simulink model "Progetto_a1_simulink_non_lineare"  (R2022b)
settings: Solver=VariableStepAuto  StartTime=0.0  StopTime=100  RelTol=1e-3
values from neighbouring files (symbols this model uses):
  DD_ampiezza = 0.3    [Progetto_a1.m]
  DD_frequenza = 0.025    [Progetto_a1.m]
  denR = deR{1}    [Progetto_a1.m]
  NN_ampiezza = 0.2    [Progetto_a1.m]
  NN_frequenza = 1e3    (= 1000)    [Progetto_a1.m]
  numR = nuR{1}    [Progetto_a1.m]
  u_e = 2.17    [Progetto_a1.m]
  WW = 2    [Progetto_a1.m]
  x = [1,2,3,4]    [Progetto_a1.m]
  x01 = theta_e    (= 1.0471975512)    [Progetto_a1.m]
  x02 = 0    [Progetto_a1.m]
  ye = x01    (= 1.0471975512)    [Progetto_a1.m]
settings Model: Creator=anton  LastModifiedBy=anton

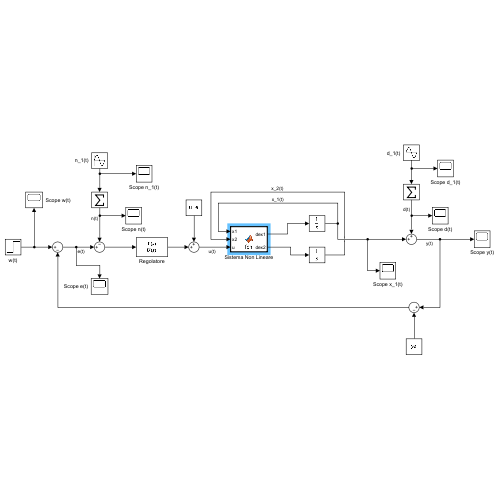
[thumbnail: Simulink's stored preview of the top-level diagram]
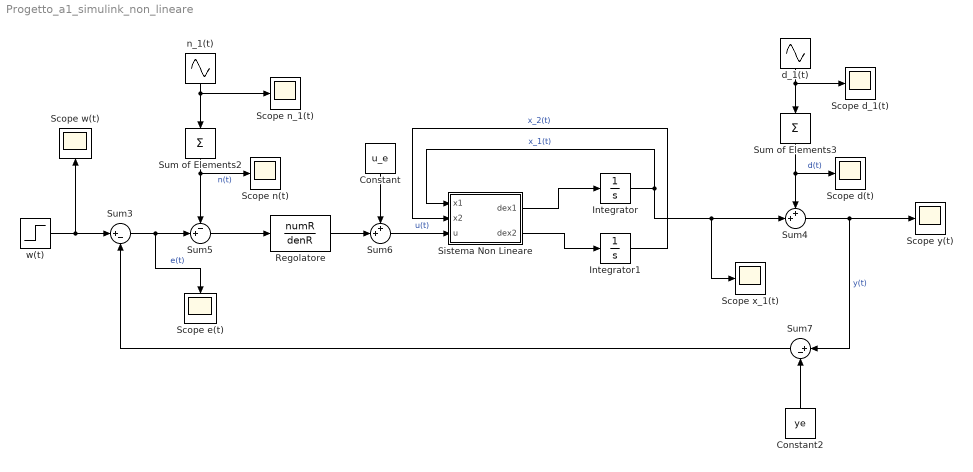
== system Progetto_a1_simulink_non_lineare ==
  Constant : Constant  Value=u_e
  Constant2 : Constant  Value=ye
  Integrator : Integrator  InitialCondition=x01
  Integrator1 : Integrator  InitialCondition=x02
  Regolatore : TransferFcn  Numerator=numR  Denominator=denR
  Scope d(t) : Scope
  Scope d_1(t) : Scope
  Scope e(t) : Scope
  Scope n(t) : Scope
  Scope n_1(t) : Scope
  Scope w(t) : Scope
  Scope x_1(t) : Scope
  Scope y(t) : Scope
  Sistema Non Lineare : MATLAB Function  TreatAsAtomicUnit=on
  Sum of Elements2 : Sum  Inputs=+  CollapseDim=4
  Sum of Elements3 : Sum  Inputs=+  CollapseDim=4
  Sum3 : Sum  Inputs=|+-
  Sum4 : Sum  Inputs=++|
  Sum5 : Sum  Inputs=-+|
  Sum6 : Sum  Inputs=++|
  Sum7 : Sum  Inputs=|+-
  d_1(t) : Sin  Amplitude=DD_ampiezza  Frequency=DD_frequenza*x  SampleTime=0
  n_1(t) : Sin  Amplitude=NN_ampiezza  Frequency=NN_frequenza*x  SampleTime=0
  w(t) : Step  Time=0  After=WW  SampleTime=0
  wires:
  Sistema Non Lineare/1(dex1) -> Integrator/1
  Sistema Non Lineare/2(dex2) -> Integrator1/1
  Integrator/1 -> Sistema Non Lineare/1(x1), Sum4/2, Scope x_1(t)/1  "x_1(t)"
  Integrator1/1 -> Sistema Non Lineare/2(x2)  "x_2(t)"
  Sum6/1 -> Sistema Non Lineare/3(u)  "u(t)"
  Constant/1 -> Sum6/1
  Regolatore/1 -> Sum6/2
  Sum of Elements2/1 -> Sum5/1, Scope n(t)/1  "n(t)"
  Sum7/1 -> Sum3/2
  Sum5/1 -> Regolatore/1
  n_1(t)/1 -> Sum of Elements2/1, Scope n_1(t)/1
  Sum3/1 -> Scope e(t)/1, Sum5/2  "e(t)"
  w(t)/1 -> Scope w(t)/1, Sum3/1
  Constant2/1 -> Sum7/2
  Sum4/1 -> Scope y(t)/1, Sum7/1  "y(t)"
  d_1(t)/1 -> Sum of Elements3/1, Scope d_1(t)/1
  Sum of Elements3/1 -> Sum4/1, Scope d(t)/1  "d(t)"

== matlab function Progetto_a1_simulink_non_lineare/Sistema Non Lineare ==
  data: x1 input; x2 input; u input; dex1 output; dex2 output
function [dex1,dex2] = fcn(x1,x2,u)
% Parametri
beta = 0.5;
J = 10;
a = 0.01;
F_v = -5;

%Sistema
dex1 = x2;
dex2 = (-beta/J)*x2+(a/(2*J))*sin(x1)*F_v+(a/J)*u;
